simulink model "Project_1_stimulinkfile"  (R2020b)
settings: Solver=VariableStepAuto  StartTime=0.0  StopTime=1  MaxStep=0.001  MinStep=0.001  RelTol=1e-4
libraries: simulink x1
settings Model: Creator=sinha  LastModifiedBy=sinha

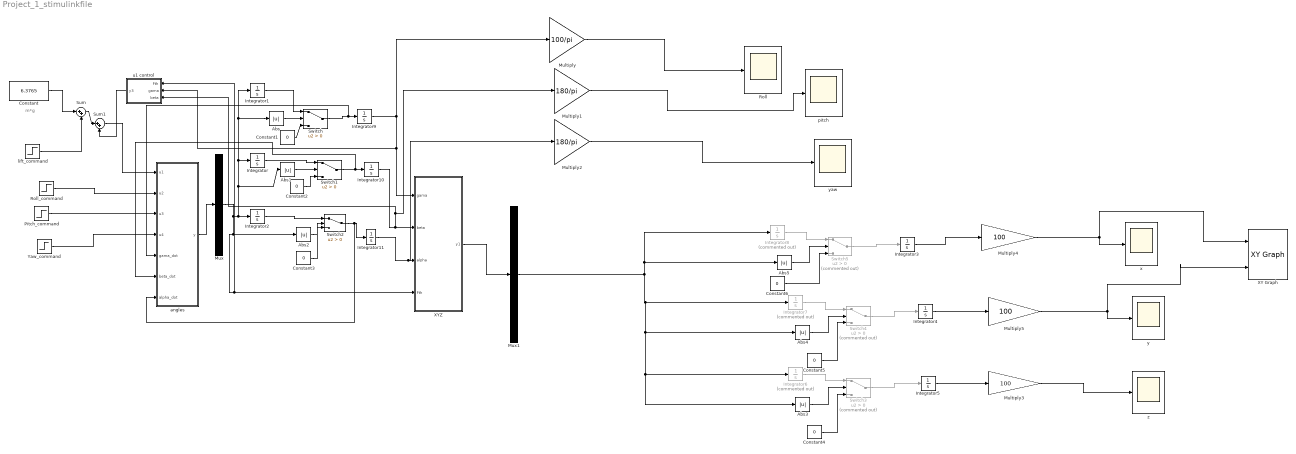
== system Project_1_stimulinkfile ==
  note: m*g
  Abs{,1..5} (6 alike) : Abs
  Constant : Constant  Value=6.3765
  Constant{1..6} (6 alike) : Constant  Value=0
  Integrator{,1..5,9..11} (9 alike) : Integrator
  Integrator6 : Integrator  Commented=on
  Integrator7 : Integrator  Commented=on
  Integrator8 : Integrator  Commented=on
  Multiply : Gain  Gain=100/pi
  Multiply1 : Gain  Gain=180/pi
  Multiply2 : Gain  Gain=180/pi
  Multiply3 : Gain  Gain=100
  Multiply4 : Gain  Gain=100
  Multiply5 : Gain  Gain=100
  Mux : Mux  Inputs=1
  Mux1 : Mux  Inputs=1
  Pitch_command : Step  Time=0.33  Before=0.5  After=0  SampleTime=0
  Roll : Scope
  Roll_command : Step  Time=0.33  Before=0.5  After=0  SampleTime=0
  Sum : Sum  Inputs=|++
  Sum1 : Sum  Inputs=|++
  Switch : Switch  Criteria=u2 > Threshold
  Switch1 : Switch  Criteria=u2 > Threshold
  Switch2 : Switch  Criteria=u2 > Threshold
  Switch3 : Switch  Commented=on  Criteria=u2 > Threshold
  Switch4 : Switch  Commented=on  Criteria=u2 > Threshold
  Switch5 : Switch  Commented=on  Criteria=u2 > Threshold
  XY Graph : simulink/Sinks/XY Graph  xmin=-1  xmax=1  ymin=-1  ymax=1  st=-1
  XYZ : MATLAB Function  TreatAsAtomicUnit=on
  Yaw_command : Step  Time=0.25  After=0  SampleTime=0
  angles : MATLAB Function  TreatAsAtomicUnit=on
  lift_command : Step  After=0  SampleTime=0
  pitch : Scope
  u1 control : MATLAB Function  TreatAsAtomicUnit=on
  x : Scope
  y : Scope
  yaw : Scope
  z : Scope
  wires:
  Constant2/1 -> Switch1/3
  Constant3/1 -> Switch2/3
  Constant1/1 -> Switch/3
  Abs/1 -> Switch/2
  Abs1/1 -> Switch1/2
  Abs2/1 -> Switch2/2
  Integrator1/1 -> Switch/1
  Integrator/1 -> Switch1/1
  Integrator2/1 -> Switch2/1
  angles/1(y) -> Mux/1
  lift_command/1 -> Sum/2
  Mux/1 -> Abs2/1, u1 control/1(Fth), XYZ/4(Fth), Abs1/1, Abs/1, Integrator1/1, Integrator/1, Integrator2/1
  Constant/1 -> Sum/1
  Sum/1 -> Sum1/1
  u1 control/1(y3) -> Sum1/2
  XYZ/1(y1) -> Mux1/1
  Multiply/1 -> Roll/1
  Multiply1/1 -> pitch/1
  Multiply2/1 -> yaw/1
  Multiply4/1 -> x/1, XY Graph/1
  Multiply5/1 -> y/1, XY Graph/2
  Multiply3/1 -> z/1
  Integrator3/1 -> Multiply4/1
  Integrator4/1 -> Multiply5/1
  Integrator5/1 -> Multiply3/1
  Switch3/1 -> Integrator5/1
  Abs3/1 -> Switch3/2
  Constant4/1 -> Switch3/3
  Integrator6/1 -> Switch3/1
  Constant5/1 -> Switch4/3
  Integrator7/1 -> Switch4/1
  Abs4/1 -> Switch4/2
  Switch4/1 -> Integrator4/1
  Constant6/1 -> Switch5/3
  Integrator8/1 -> Switch5/1
  Abs5/1 -> Switch5/2
  Switch5/1 -> Integrator3/1
  Mux1/1 -> Integrator8/1, Abs5/1, Abs3/1, Integrator6/1, Abs4/1, Integrator7/1
  Switch/1 -> angles/5(gama_dot), Integrator9/1
  Switch1/1 -> angles/6(beta_dot), Integrator10/1
  Switch2/1 -> angles/7(alpha_dot), Integrator11/1
  Integrator9/1 -> XYZ/1(gama), u1 control/2(gama), Multiply/1
  Integrator10/1 -> Multiply1/1, u1 control/3(beta), XYZ/2(beta)
  Integrator11/1 -> Multiply2/1, XYZ/3(alpha)
  Roll_command/1 -> angles/2(u2)
  Pitch_command/1 -> angles/3(u3)
  Yaw_command/1 -> angles/4(u4)
  Sum1/1 -> angles/1(u1)

== matlab function Project_1_stimulinkfile/u1 control ==
  data: Fth input; y3 output; gama input; beta input
function y3 = fcn(Fth,gama,beta)%#codegen
du1=Fth*(1-(cos(gama)*cos(beta)));
y3 = du1;

== matlab function Project_1_stimulinkfile/angles ==
  data: u1 input; y output; u2 input; u3 input; u4 input; gama_dot input; beta_dot input; alpha_dot input
function y = fcn(u1,u2,u3,u4,gama_dot,beta_dot,alpha_dot)%#codegen
Ixx=7.5e-3;
Iyy=7.5e-3; 
Izz=1.3e-2;
L=0.23;
Jr=6e-5;
km=7.5e-7;
kf=3.13e-5;
omega1_sq=((0.25/kf)*u1+(0.5/kf)*u3-(0.25/km)*u4);
omega1=sqrt(abs(omega1_sq));
omega2_sq=((0.25/kf)*u1-(0.5/kf)*u3-(0.25/km)*u4);
omega2=sqrt(abs(omega2_sq));
omega3_sq=((0.25/kf)*u1-(0.5/kf)*u2+(0.25/km)*u4);
omega3=sqrt(abs(omega3_sq));
omega4_sq=((0.25/kf)*u1+(0.5/kf)*u2+(0.25/km)*u4);
omega4=sqrt(abs(omega4_sq));
F1=kf*omega1_sq;F2=kf*omega2_sq;F3=kf*omega3_sq;F4=kf*omega4_sq; %force of each propeller
Fth=(F1+F2+F3+F4);  %lift force
Mb=[L*u2;L*u3;u4];  %moments for roll, pitch and yaw
omegar=omega1+omega2-omega3-omega4;
gama_ddot=(1/Ixx)*((-beta_dot*(Izz-Iyy)*alpha_dot)-(beta_dot*Jr*omegar)+Mb(1));
beta_ddot=(1/Iyy)*((-alpha_dot*(Ixx-Izz)*gama_dot)+(gama_dot*Jr*omegar)+Mb(2));
alpha_ddot=(1/Izz)*((-beta_dot*(Iyy-Ixx)*gama_dot)+Mb(3));
disp(gama_ddot);
y = [gama_ddot beta_ddot alpha_ddot, Fth];
end

== matlab function Project_1_stimulinkfile/XYZ ==
  data: gama input; y1 output; beta input; alpha input; Fth input
function y1= fcn(gama,beta,alpha,Fth)
%#codegen
m=0.65;g=9.81;
    x_ddot= -(Fth/m).*((cos(gama).*sin(beta).*cos(alpha))+(sin(gama).*sin(alpha)));
    y_ddot= -(Fth/m).*((cos(gama).*sin(beta).*sin(alpha))-(sin(gama).*cos(alpha)));  
    z_ddot= g-(Fth/m).*(cos(gama).*cos(beta));
y1 = [x_ddot y_ddot z_ddot];
end
